simulink model "Tf"  (R2025b)
settings: Solver=VariableStepAuto  StartTime=0.0  StopTime=20  RelTol=1e-3
values from neighbouring files (symbols this model uses):
  Kp = vetKp(i)    [LabControle.m]
  Ti = vetTi(j)    [LabControle.m]
settings Model: Creator=Pato

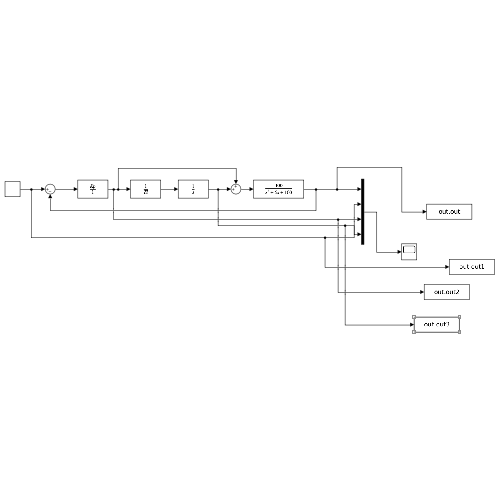
[thumbnail: Simulink's stored preview of the top-level diagram]
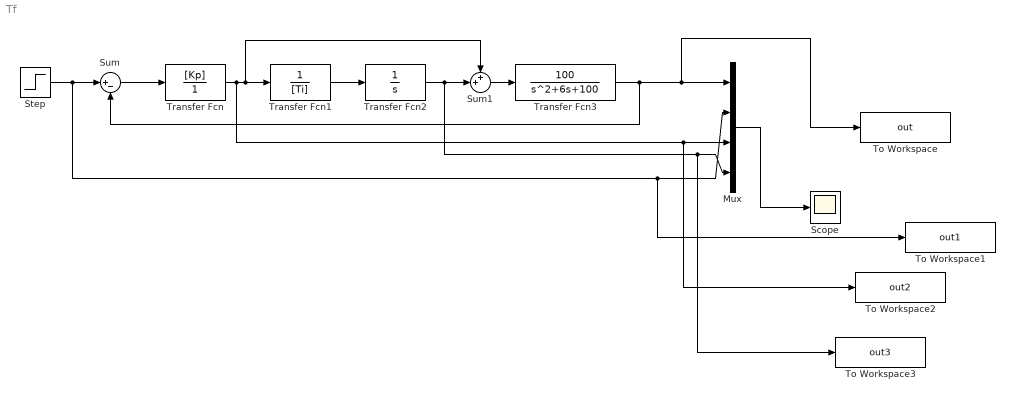
== system Tf ==
  Mux : Mux
  Scope : Scope
      settings: ActiveDisplayYMinimum=-0.6644585870417643  ActiveDisplayYMaximum=2.781107030339145
  Step : Step  SampleTime=0.01
  Sum : Sum  Inputs=|+-
  Sum1 : Sum  Inputs=++|
  To Workspace : ToWorkspace  VariableName=out  SaveFormat=Timeseries  SampleTime=-1
  To Workspace1 : ToWorkspace  VariableName=out1  SaveFormat=Timeseries  SampleTime=-1
  To Workspace2 : ToWorkspace  VariableName=out2  SaveFormat=Timeseries  SampleTime=-1
  To Workspace3 : ToWorkspace  VariableName=out3  SaveFormat=Timeseries  SampleTime=-1
  Transfer Fcn : TransferFcn  Numerator=[Kp]  Denominator=1
  Transfer Fcn1 : TransferFcn  Denominator=[Ti]
  Transfer Fcn2 : TransferFcn  Denominator=[1 0]
  Transfer Fcn3 : TransferFcn  Numerator=[100]  Denominator=[1 6 100]
  wires:
  Transfer Fcn2/1 -> To Workspace3/1, Mux/4, Sum1/2
  Sum1/1 -> Transfer Fcn3/1
  Step/1 -> To Workspace1/1, Mux/2, Sum/1
  Transfer Fcn3/1 -> To Workspace/1, Mux/1, Sum/2
  Transfer Fcn1/1 -> Transfer Fcn2/1
  Transfer Fcn/1 -> To Workspace2/1, Mux/3, Sum1/1, Transfer Fcn1/1
  Sum/1 -> Transfer Fcn/1
  Mux/1 -> Scope/1
